simulink model "openLoop_inputFromFile"  (Simulink 8.9)
settings: Solver=ode45  StartTime=0.0  StopTime=max(t)  RelTol=1e-3  EnableMultiTasking=on
undefined symbols (not defined in the file or in its folder): isCurrent
libraries: cjt_library_models x1
settings Model: SuppressorTable=22 serialization::archive 11 0 6 0 0 0 11 0  Creator=joern  LastModifiedBy=wesley
settings DataIOCC: SignalLoggingSaveFormat=Dataset
settings DebuggingCC: UnderspecifiedInitializationDetection=Simplified  MergeDetectMultiDrivingBlocksExec=error  SolverPrmCheckMsg=warning  FcnCallInpInsideContextMsg=error  AllowSymbolicDim=off  StateNameClashWarn=none
settings GRTTargetCC: CombineOutputUpdateFcns=on  GRTInterface=off

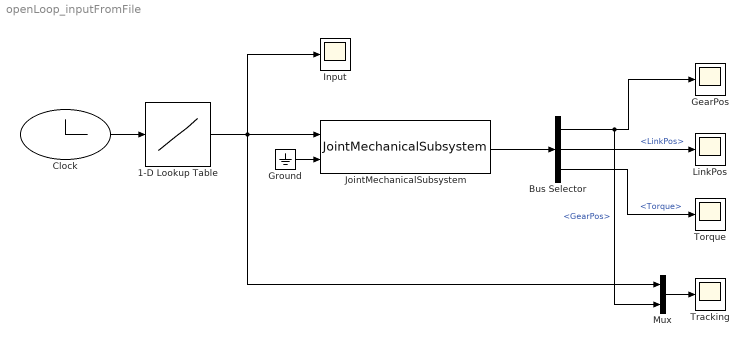
== system openLoop_inputFromFile ==
  1-D Lookup Table : Lookup_n-D  NumberOfTableDimensions=1  BreakpointsSpecification=Even spacing  BreakpointsForDimension1Spacing=1e-3  Table=isCurrent  InternalRulePriority=Speed  RndMeth=Simplest  InputSameDT=on
  Bus Selector : BusSelector  OutputSignals=GearPos,LinkPos,Torque
  Clock : Clock
  GearPos : Scope
  Ground : Ground
  Input : Scope
  JointMechanicalSubsystem : cjt_library_models/Joint models/JointMechanicalSubsystem  jointObj=jointObj  fc_vel=499  fc_torque=499  input_delay=1  output_delay=1  quantize=on  quantize_bits=19  input_noise_enabled=off  output_noise_enabled=off  var_u=0.12^2  var_y=1.8e-10
  LinkPos : Scope
  Mux : Mux  Inputs=2
  Torque : Scope
  Tracking : Scope
  wires:
  JointMechanicalSubsystem/1 -> Bus Selector/1
  Bus Selector/2 -> LinkPos/1  "<LinkPos>"
  Bus Selector/3 -> Torque/1  "<Torque>"
  Mux/1 -> Tracking/1
  Bus Selector/1 -> Mux/2, GearPos/1  "<GearPos>"
  1-D Lookup Table/1 -> JointMechanicalSubsystem/1, Input/1, Mux/1
  Clock/1 -> 1-D Lookup Table/1
  Ground/1 -> JointMechanicalSubsystem/2
